simulink model "SIM_EXP8"  (R2022a)
settings: Solver=VariableStepAuto  StartTime=0.0  StopTime=5  MaxStep=0.01  RelTol=1e-3
settings Model: Creator=Dell  LastModifiedBy=Dell

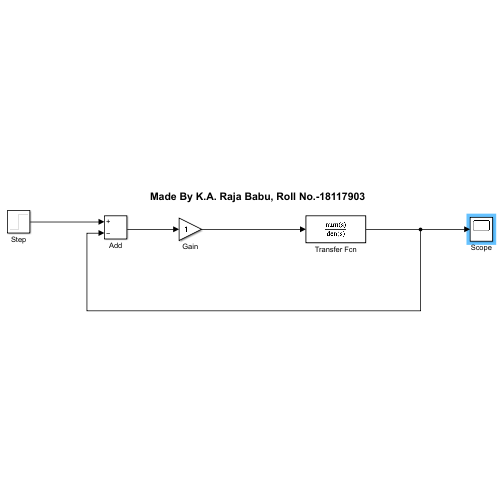
[thumbnail: Simulink's stored preview of the top-level diagram]
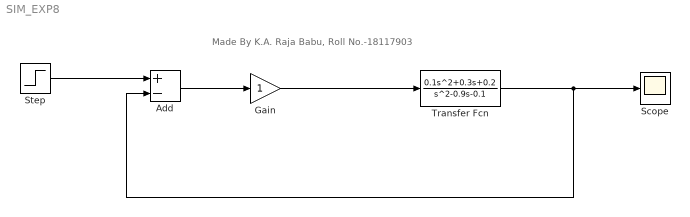
== system SIM_EXP8 ==
  note: Made By K.A. Raja Babu, Roll No.-18117903
  Add : Sum  Inputs=+-
  Gain : Gain
  Scope : Scope
  Step : Step  Before=1  SampleTime=0
  Transfer Fcn : TransferFcn  Numerator=[0.1 0.3 0.2]  Denominator=[1 -0.9 -0.1]
  wires:
  Step/1 -> Add/1
  Add/1 -> Gain/1
  Gain/1 -> Transfer Fcn/1
  Transfer Fcn/1 -> Add/2, Scope/1
